simulink model "TST_FuelT_VD"  (R2016b)
settings: Solver=FixedStepDiscrete  StartTime=0.0  StopTime=simTime  FixedStep=sampleTime  RelTol=1e-3
values from neighbouring files (symbols this model uses):
  testCase = 1    [initTST_FuelT_VD_001.m]    (also in initTST_FuelT_VD_002.m = 2; initTST_FuelT_VD_003.m = 3)
libraries: simulink x5, UnitTest_Lib x3
settings Model: Creator=dulinggang  LastModifiedBy=dulinggang
settings DebuggingCC: SignalRangeChecking=error

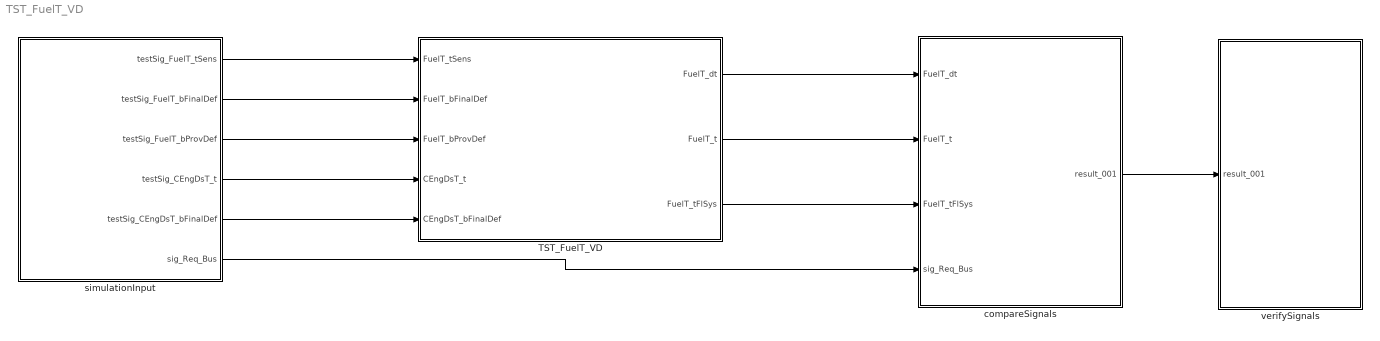
== system TST_FuelT_VD ==
  TST_FuelT_VD : Subsystem
  compareSignals : Subsystem
  simulationInput : Subsystem
  verifySignals : Subsystem
  wires:
  simulationInput/1(testSig_FuelT_tSens) -> TST_FuelT_VD/1(FuelT_tSens)
  simulationInput/2(testSig_FuelT_bFinalDef) -> TST_FuelT_VD/2(FuelT_bFinalDef)
  simulationInput/3(testSig_FuelT_bProvDef) -> TST_FuelT_VD/3(FuelT_bProvDef)
  simulationInput/4(testSig_CEngDsT_t) -> TST_FuelT_VD/4(CEngDsT_t)
  simulationInput/5(testSig_CEngDsT_bFinalDef) -> TST_FuelT_VD/5(CEngDsT_bFinalDef)
  TST_FuelT_VD/1(FuelT_dt) -> compareSignals/1(FuelT_dt)
  TST_FuelT_VD/2(FuelT_t) -> compareSignals/2(FuelT_t)
  TST_FuelT_VD/3(FuelT_tFlSys) -> compareSignals/3(FuelT_tFlSys)
  simulationInput/6(sig_Req_Bus) -> compareSignals/4(sig_Req_Bus)
  compareSignals/1(result_001) -> verifySignals/1(result_001)

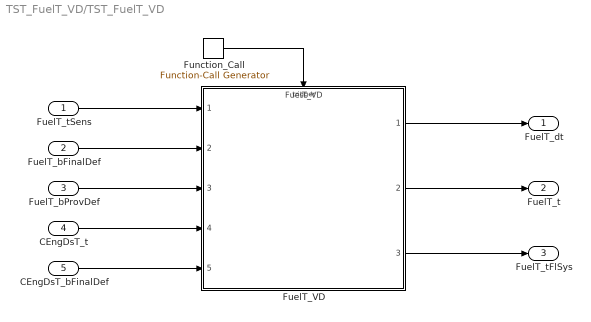
== system TST_FuelT_VD/TST_FuelT_VD ==
  FuelT_tSens : Inport
  FuelT_bFinalDef : Inport  Port=2
  FuelT_bProvDef : Inport  Port=3
  CEngDsT_t : Inport  Port=4
  CEngDsT_bFinalDef : Inport  Port=5
  FuelT_VD : ModelReference  ModelNameDialog=FuelT_VD  SimulationMode=Normal  ModelReferenceVersion=1.36  TriggerPortName=function  TriggerPortTriggerType=function-call  TriggerPortStatesWhenEnabling=held
  Function_Call : simulink/Ports & Subsystems/Function-Call Generator  sample_time=sampleTime  numberOfIterations=1
  FuelT_dt : Outport
  FuelT_t : Outport  Port=2
  FuelT_tFlSys : Outport  Port=3
  wires:
  Function_Call/1 -> FuelT_VD/Trigger
  FuelT_tSens/1 -> FuelT_VD/1
  FuelT_bFinalDef/1 -> FuelT_VD/2
  FuelT_bProvDef/1 -> FuelT_VD/3
  CEngDsT_t/1 -> FuelT_VD/4
  CEngDsT_bFinalDef/1 -> FuelT_VD/5
  FuelT_VD/1 -> FuelT_dt/1
  FuelT_VD/2 -> FuelT_t/1
  FuelT_VD/3 -> FuelT_tFlSys/1

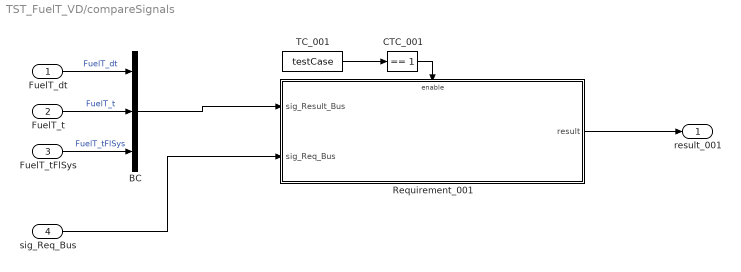
== system TST_FuelT_VD/compareSignals ==
  FuelT_dt : Inport
  FuelT_t : Inport  Port=2
  FuelT_tFlSys : Inport  Port=3
  sig_Req_Bus : Inport  Port=4
  BC : BusCreator  Inputs=3
  CTC_001 : simulink/Logic and Bit Operations/Compare To Constant  relop===  const=1  OutDataTypeStr=boolean
  Requirement_001 : Subsystem
  TC_001 : Constant  Value=testCase
  result_001 : Outport
  wires:
  FuelT_dt/1 -> BC/1  "FuelT_dt"
  FuelT_t/1 -> BC/2  "FuelT_t"
  FuelT_tFlSys/1 -> BC/3  "FuelT_tFlSys"
  TC_001/1 -> CTC_001/1
  CTC_001/1 -> Requirement_001/Enable
  sig_Req_Bus/1 -> Requirement_001/2(sig_Req_Bus)
  BC/1 -> Requirement_001/1(sig_Result_Bus)
  Requirement_001/1(result) -> result_001/1

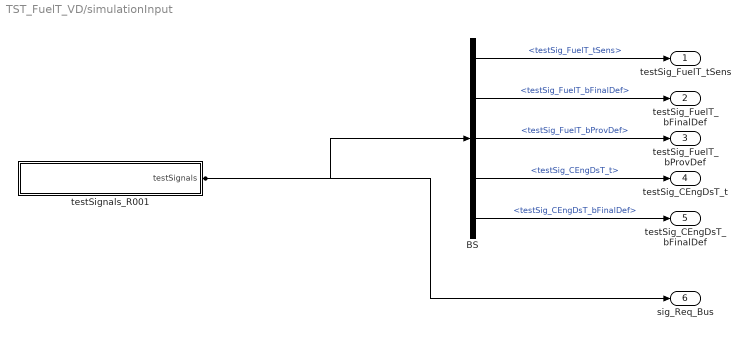
== system TST_FuelT_VD/simulationInput ==
  BS : BusSelector  OutputSignals=testSig_FuelT_tSens,testSig_FuelT_bFinalDef,testSig_FuelT_bProvDef,testSig_CEngDsT_t,testSig_CEngDsT_bFinalDef
  testSignals_R001 : Subsystem
  testSig_FuelT_tSens : Outport
  testSig_FuelT_bFinalDef : Outport  Port=2
  testSig_FuelT_bProvDef : Outport  Port=3
  testSig_CEngDsT_t : Outport  Port=4
  testSig_CEngDsT_bFinalDef : Outport  Port=5
  sig_Req_Bus : Outport  Port=6
  wires:
  BS/1 -> testSig_FuelT_tSens/1  "<testSig_FuelT_tSens>"
  BS/2 -> testSig_FuelT_bFinalDef/1  "<testSig_FuelT_bFinalDef>"
  BS/3 -> testSig_FuelT_bProvDef/1  "<testSig_FuelT_bProvDef>"
  BS/4 -> testSig_CEngDsT_t/1  "<testSig_CEngDsT_t>"
  BS/5 -> testSig_CEngDsT_bFinalDef/1  "<testSig_CEngDsT_bFinalDef>"
  testSignals_R001/1(testSignals) -> BS/1, sig_Req_Bus/1

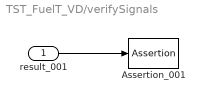
== system TST_FuelT_VD/verifySignals ==
  result_001 : Inport
  Assertion_001 : Assertion  Enabled=off
  wires:
  result_001/1 -> Assertion_001/1

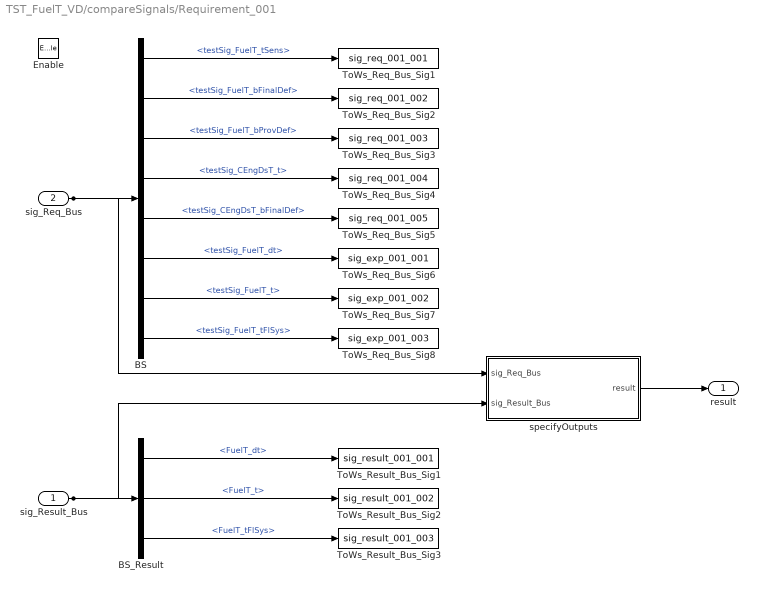
== system TST_FuelT_VD/compareSignals/Requirement_001 ==
  sig_Result_Bus : Inport
  sig_Req_Bus : Inport  Port=2
  Enable : EnablePort
  BS : BusSelector  OutputSignals=testSig_FuelT_tSens,testSig_FuelT_bFinalDef,testSig_FuelT_bProvDef,testSig_CEngDsT_t,testSig_CEngDsT_bFinalDef,testSig_FuelT_dt,testSig_FuelT_t,testSig_FuelT_tFlSys
  BS_Result : BusSelector  OutputSignals=FuelT_dt,FuelT_t,FuelT_tFlSys
  ToWs_Req_Bus_Sig1 : ToWorkspace  VariableName=sig_req_001_001  SaveFormat=Structure With Time
  ToWs_Req_Bus_Sig2 : ToWorkspace  VariableName=sig_req_001_002  SaveFormat=Structure With Time
  ToWs_Req_Bus_Sig3 : ToWorkspace  VariableName=sig_req_001_003  SaveFormat=Structure With Time
  ToWs_Req_Bus_Sig4 : ToWorkspace  VariableName=sig_req_001_004  SaveFormat=Structure With Time
  ToWs_Req_Bus_Sig5 : ToWorkspace  VariableName=sig_req_001_005  SaveFormat=Structure With Time
  ToWs_Req_Bus_Sig6 : ToWorkspace  VariableName=sig_exp_001_001  SaveFormat=Structure With Time
  ToWs_Req_Bus_Sig7 : ToWorkspace  VariableName=sig_exp_001_002  SaveFormat=Structure With Time
  ToWs_Req_Bus_Sig8 : ToWorkspace  VariableName=sig_exp_001_003  SaveFormat=Structure With Time
  ToWs_Result_Bus_Sig1 : ToWorkspace  VariableName=sig_result_001_001  SaveFormat=Structure With Time
  ToWs_Result_Bus_Sig2 : ToWorkspace  VariableName=sig_result_001_002  SaveFormat=Structure With Time
  ToWs_Result_Bus_Sig3 : ToWorkspace  VariableName=sig_result_001_003  SaveFormat=Structure With Time
  specifyOutputs : Subsystem
  result : Outport
  wires:
  sig_Req_Bus/1 -> BS/1, specifyOutputs/1(sig_Req_Bus)
  BS/1 -> ToWs_Req_Bus_Sig1/1  "<testSig_FuelT_tSens>"
  BS/2 -> ToWs_Req_Bus_Sig2/1  "<testSig_FuelT_bFinalDef>"
  BS/3 -> ToWs_Req_Bus_Sig3/1  "<testSig_FuelT_bProvDef>"
  BS/4 -> ToWs_Req_Bus_Sig4/1  "<testSig_CEngDsT_t>"
  BS/5 -> ToWs_Req_Bus_Sig5/1  "<testSig_CEngDsT_bFinalDef>"
  BS/6 -> ToWs_Req_Bus_Sig6/1  "<testSig_FuelT_dt>"
  BS/7 -> ToWs_Req_Bus_Sig7/1  "<testSig_FuelT_t>"
  BS/8 -> ToWs_Req_Bus_Sig8/1  "<testSig_FuelT_tFlSys>"
  sig_Result_Bus/1 -> BS_Result/1, specifyOutputs/2(sig_Result_Bus)
  BS_Result/1 -> ToWs_Result_Bus_Sig1/1  "<FuelT_dt>"
  BS_Result/2 -> ToWs_Result_Bus_Sig2/1  "<FuelT_t>"
  BS_Result/3 -> ToWs_Result_Bus_Sig3/1  "<FuelT_tFlSys>"
  specifyOutputs/1(result) -> result/1

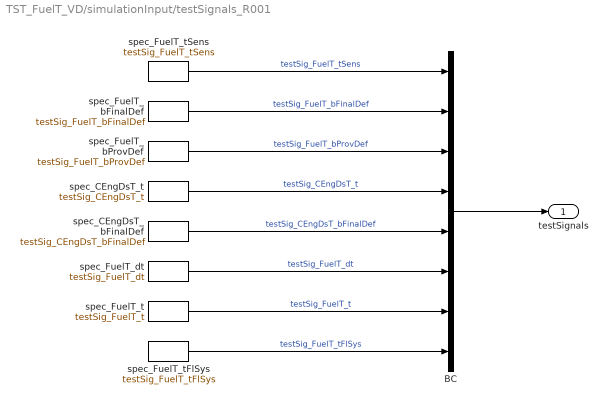
== system TST_FuelT_VD/simulationInput/testSignals_R001 ==
  BC : BusCreator  Inputs=8
  spec_CEngDsT_bFinalDef : FromWorkspace  VariableName=testSig_CEngDsT_bFinalDef  Interpolate=off  OutputAfterFinalValue=Holding final value
  spec_CEngDsT_t : FromWorkspace  VariableName=testSig_CEngDsT_t  Interpolate=off  OutputAfterFinalValue=Holding final value
  spec_FuelT_bFinalDef : FromWorkspace  VariableName=testSig_FuelT_bFinalDef  Interpolate=off  OutputAfterFinalValue=Holding final value
  spec_FuelT_bProvDef : FromWorkspace  VariableName=testSig_FuelT_bProvDef  Interpolate=off  OutputAfterFinalValue=Holding final value
  spec_FuelT_dt : FromWorkspace  VariableName=testSig_FuelT_dt  Interpolate=off  OutputAfterFinalValue=Holding final value
  spec_FuelT_t : FromWorkspace  VariableName=testSig_FuelT_t  Interpolate=off  OutputAfterFinalValue=Holding final value
  spec_FuelT_tFlSys : FromWorkspace  VariableName=testSig_FuelT_tFlSys  Interpolate=off  OutputAfterFinalValue=Holding final value
  spec_FuelT_tSens : FromWorkspace  VariableName=testSig_FuelT_tSens  Interpolate=off  OutputAfterFinalValue=Holding final value
  testSignals : Outport
  wires:
  BC/1 -> testSignals/1
  spec_FuelT_tSens/1 -> BC/1  "testSig_FuelT_tSens"
  spec_FuelT_bFinalDef/1 -> BC/2  "testSig_FuelT_bFinalDef"
  spec_FuelT_bProvDef/1 -> BC/3  "testSig_FuelT_bProvDef"
  spec_CEngDsT_t/1 -> BC/4  "testSig_CEngDsT_t"
  spec_CEngDsT_bFinalDef/1 -> BC/5  "testSig_CEngDsT_bFinalDef"
  spec_FuelT_dt/1 -> BC/6  "testSig_FuelT_dt"
  spec_FuelT_t/1 -> BC/7  "testSig_FuelT_t"
  spec_FuelT_tFlSys/1 -> BC/8  "testSig_FuelT_tFlSys"

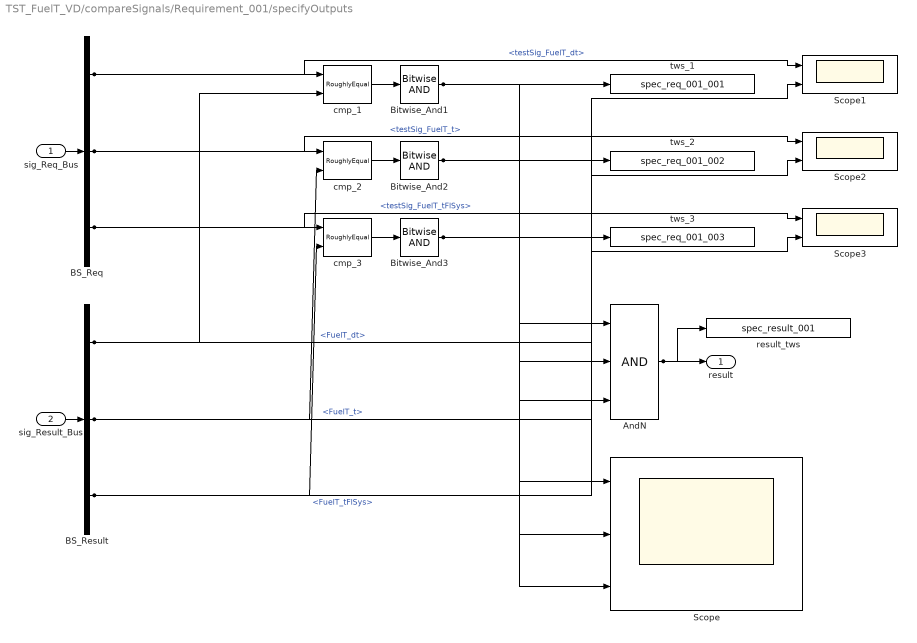
== system TST_FuelT_VD/compareSignals/Requirement_001/specifyOutputs ==
  sig_Req_Bus : Inport
  sig_Result_Bus : Inport  Port=2
  AndN : Logic  Inputs=3
  BS_Req : BusSelector  OutputSignals=testSig_FuelT_dt,testSig_FuelT_t,testSig_FuelT_tFlSys
  BS_Result : BusSelector  OutputSignals=FuelT_dt,FuelT_t,FuelT_tFlSys
  Bitwise_And1 : simulink/Logic and Bit Operations/Bitwise Operator  logicop=AND  UseBitMask=off  BitMask=bin2dec('11011001')  BitMaskRealWorld=Stored Integer
  Bitwise_And2 : simulink/Logic and Bit Operations/Bitwise Operator  logicop=AND  UseBitMask=off  BitMask=bin2dec('11011001')  BitMaskRealWorld=Stored Integer
  Bitwise_And3 : simulink/Logic and Bit Operations/Bitwise Operator  logicop=AND  UseBitMask=off  BitMask=bin2dec('11011001')  BitMaskRealWorld=Stored Integer
  Scope : Scope  NumInputPorts=3
  Scope1 : Scope  NumInputPorts=2
  Scope2 : Scope  NumInputPorts=2
  Scope3 : Scope  NumInputPorts=2
  cmp_1 : UnitTest_Lib/RoughlyEqual  slope=0.1
  cmp_2 : UnitTest_Lib/RoughlyEqual  slope=0.1
  cmp_3 : UnitTest_Lib/RoughlyEqual  slope=0.1
  result_tws : ToWorkspace  VariableName=spec_result_001
  tws_1 : ToWorkspace  VariableName=spec_req_001_001
  tws_2 : ToWorkspace  VariableName=spec_req_001_002
  tws_3 : ToWorkspace  VariableName=spec_req_001_003
  result : Outport
  wires:
  sig_Req_Bus/1 -> BS_Req/1
  sig_Result_Bus/1 -> BS_Result/1
  AndN/1 -> result/1, result_tws/1
  BS_Req/1 -> cmp_1/1, Scope1/1  "<testSig_FuelT_dt>"
  BS_Result/1 -> cmp_1/2, Scope1/2  "<FuelT_dt>"
  cmp_1/1 -> Bitwise_And1/1
  Bitwise_And1/1 -> tws_1/1, AndN/1, Scope/1
  BS_Req/2 -> cmp_2/1, Scope2/1  "<testSig_FuelT_t>"
  BS_Result/2 -> cmp_2/2, Scope2/2  "<FuelT_t>"
  cmp_2/1 -> Bitwise_And2/1
  Bitwise_And2/1 -> tws_2/1, AndN/2, Scope/2
  BS_Req/3 -> cmp_3/1, Scope3/1  "<testSig_FuelT_tFlSys>"
  BS_Result/3 -> cmp_3/2, Scope3/2  "<FuelT_tFlSys>"
  cmp_3/1 -> Bitwise_And3/1
  Bitwise_And3/1 -> tws_3/1, AndN/3, Scope/3
